simulink model "ds_modelica_weather"  (R2020a)
settings: Solver=ode1  StartTime=0.0  StopTime=Inf  FixedStep=0.001  RelTol=1e-3
PostLoadFcn:
  | if any(exist('dsrtsu_mdlpostloadfcn', 'file') ~= 0), dsrtsu_mdlpostloadfcn('Execute', bdroot); end
InitFcn:
  | , if any(exist('rtifpga_mdlclblib', 'file') ~= 0), rtifpga_mdlclblib('Init', bdroot); end,
  | , if any(exist('dsmpb_private', 'file') ~= 0), dsmpb_private('dsmpb_mdlclblib', 'Init', bdroot); end,
libraries: dsmpblib x1
PreSaveFcn:
  | , if any(exist('dsmpb_private', 'file') ~= 0), dsmpb_private('dsmpb_mdlclblib', 'PreSave', bdroot); end,
CloseFcn:
  | , if any(exist('dsmpb_private', 'file') ~= 0), dsmpb_private('dsmpb_mdlclblib', 'Close', bdroot); end,
settings Model: RTICANMMDATA=struct('GeneralSetupData',struct('modelroot','D:\github\dspace-modelica-example\dSpaceExample','generalsettings',struct('filesettings',struct('destfolder',struct('Name','RTICANMM_FILES','Check',1),'buildfolder',struct('Name','.','Check',1),'AbsDestfolder',struct('Name','D:\github\dspace-modelica-example\dSpaceExample\RTICANMM_FILES'),'AbsBuildfolder',struct('Name','D:\github\dspace-modelica-example\dSpaceExample'))),'options',struct('addpaths',1,'rmpaths',1,'addtrcexclusion',true,'cannavigator',struct('checkmonitoring',0),'show_usrtrc',0,'use_usrtrc',0),'advanced',struct('options',ones(1,100)),'MPSetup',{{}},'RTI',struct('Type','DSRT','Ver','4.3','Date','02-May-2020'),'modelname','ds_modelica_weather','block','ds_modelica_weather'))  DSRTSU_INTERNAL_RTIFPGA=160  DSMPB_ID_DATA={'121',struct('BlockId','15cad6c1-5c06-4fa3-8d72-980126a11d0f','SignalIds',{{'1464f171-9d95-458e-bcaf-80b82fdb8b87'}}),'122',struct('BlockId','3f54ef79-c7ab-4360-bc2a-717f94988ba9','SignalIds',{{'4ded6036-5f3c-446a-9a50-a2f43caa1de9'}}),'123',struct('BlockId','5b0f3eb3-8eee-4187-a879-1e3532fb32ad','SignalIds',{{'cf7abe49-a5c7-4834-bdd1-b99bcd3cf414'}}),'124',struct('BlockId','811b07df-2fcb-4c14-ad4d-f777e9630052','SignalIds',{{'eb3c2c6c-56b8-4259-a6b1-e5e06496ac5b'}}),'13',struct('BlockId','15cad6c1-5c06-4fa3-8d72-980126a11d0f','SignalIds',{{'1464f171-9d95-458e-bcaf-80b82fdb8b87'}}),'153',struct('BlockId','811b07df-2fcb-4c14-ad4d-f777e9630052','SignalIds',{{'eb3c2c6c-56b8-4259-a6b1-e5e06496ac5b'}})}  Creator=yangyang.fu  LastModifiedBy=yangyang.fu
settings OptimizationCC: BlockReduction=off  ConditionallyExecuteInputs=off  OptimizeBlockIOStorage=off  BufferReuse=off
settings DebuggingCC: TasksWithSamePriorityMsg=none
settings HardwareCC: ProdBitPerPointer=32  ProdBitPerSizeT=32  ProdBitPerPtrDiffT=32  ProdLargestAtomicInteger=Integer  ProdWordSize=32  ProdLongLongMode=on  ProdHWDeviceType=Custom Processor->Custom
settings ModelReferenceCC: EnableParallelModelReferenceBuilds=on
settings SFSimCC: MATLABDynamicMemAlloc=off
settings RTWCC: Description=dSPACE Run-Time Target (for VEOS on Windows and ConfigurationDesk)  SystemTargetFile=dsrt.tlc  GenCodeOnly=on  MakeCommand=make_dsrt  TemplateMakefile=dsrt_default_tmf  RTWVerbose=off  CustomInclude="\"C:\\Program Files\\Dymola 2021\\Source\" \"D:\\github\\dspace-modelica-example\\Libraries\\Buildings 7.0.0\\Resources\\C-Sources\""
settings STFCustomTargetCC: TargetLangStandard=C99 (ISO)  ParMdlRefBuildCompliant=on  SystemTargetFile=dsrt.tlc
settings GRTTargetCC: CompOptLevelCompliant=off  ConcurrentExecutionCompliant=off  CombineOutputUpdateFcns=off  MatFileLogging=off  CPPClassGenCompliant=off  UseToolchainInfoCompliant=off

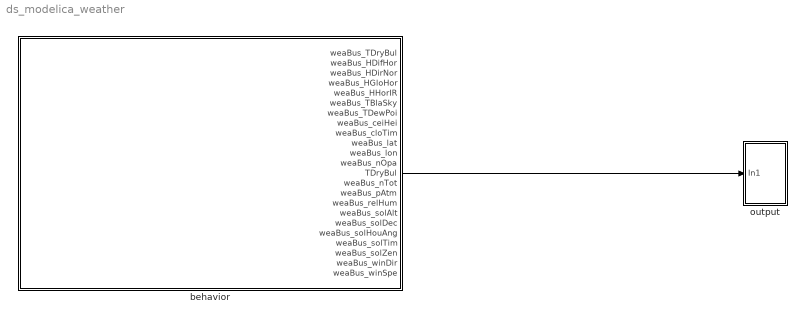
== system ds_modelica_weather ==
  behavior : Subsystem
  output : Subsystem
  wires:
  behavior/13(TDryBul) -> output/1(In1)

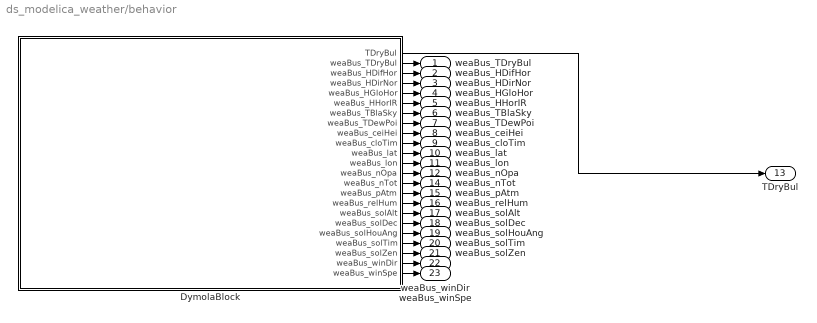
== system ds_modelica_weather/behavior ==
  DymolaBlock : Subsystem  Tag=19-Oct-2021 13:05:11#4854
      mask help:
      | Dymola block.
      | A dymola block allows acausal physical modeling.
      | See Dymola manual for usage.
      settings: CopyFcn=newDymolaGui('19-Oct-2021 13:05:11#4854','Copy');  DeleteFcn=if exist('newDymolaGui') newDymolaGui('ds_modelica_weather/behavior/DymolaBlock','Delete'); end;  NameChangeFcn=newDymolaGui('19-Oct-2021 13:05:11#4854','Copy');  OpenFcn=newDymolaGui('ds_modelica_weather/behavior/DymolaBlock','Init');
      mask Display: image(reshape([1;1;1;1;1;1;1;1;1;1;1;1;1;1;1;1;1;1;1;1;1;1;0;0;0;0;0;0;0;0;0;0;1;1;1;1;1;1;1;1;0;1;1;1;1;1;1;1;1;0;1;1;1;1;1;0;0;0;0;0;0;0;1;1;0;0;0;0;0;0;0;1;1;0;0;0;0;0;0;0;1;1;0;0;0;0;0;0;0;1;1;0;0;0;0;0;0;0;1;1;0;0;0;0;0;0;0;1;1;0;0;0;0;0;0;0;1;1;0;0;0;0;0;0;0;1;1;0;0;0;0;0;0;0;1;1;0;0;0;0;0;0;0;1;1;0;0;0;0;0;0;0;1;1;0;0;0;0;0;0;0;1;1;0;0;0;0;0;0;0;1;1;0;0;0;0;0;0;0;1;1;0;0;0;0;0;0;0;1;1;0;0;0;0;0;0;0;1;1;0;0;0;0;0;0;0;1;1;0;0;0;0;0;0;0;1;1;0;0;0;0;0;0;0;1;1;0;0;0;0;0;0;0;1;1;0;0;0;0;0;0;0;1;1;0;0;0;0;0;0;0;1;1;0;0;0;0;0;0;0;1;1;0;0;0;0;0;0;0;1;1;1;1;1;0;1;1;1;1;1;1;1;1;0;1;1;1;1;1;1;1;1;0;0;0;0;0;0;0;0;0;0;1;1;1;1;1;1;1;1;1;1;1;1;1;1;1;1;1;1;1;1;1;1;1;1;1;1;1;1;1;1;1;1;1;1;1;1;1;1;1;1;1;1;1;1;0;0;0;0;0;0;0;0;0;0;1;1;1;1;1;1;1;1;0;1;1;1;1;1;1;1;1;0;1;1;1;1;1;0;0;0;0;0;0;0;1;1;0;0;0;0;0;0;0;1;1;0;0;0;0;0;0;0;1;1;0;0;0;0;0;0;0;1;1;0;0;0;0;0;0;0;1;1;0;0;0;0;0;0;0;1;1;0;0;0;0;0;0;0;1;1;0;0;0;0;0;0;0;1;1;0;0;0;0;0;0;0;1;1;0;0;0;0;0;0;0;1;1;0;0;0;0;0;0;0;1;1;0;0;0;0;0;0;0;1;1;0;0;0;0;0;0;0;1;1;0;0;0;0;0;0;0;1;1;0;0;0;0;0;0;0;1;1;0;0;0;0;0;0;0;1;1;0;0;0;0;0;0;0;1;1;0;0;0;0;0;0;0;1;1;0;0;0;0;0;0;0;1;1;0;0;0;0;0;0;0;1;1;0;0;0;0;0;0;0;1;1;0;0;0;0;0;0;0;1;1;0;0;0;0;0;0;0;1;1;0;0;0;0;0;0;0;1;1;1;1;1;0;1;1;1;1;1;1;1;1;0;1;1;1;1;1;1;1;1;0;0;0;0;0;0;0;0;0;0;1;1;1;1;1;1;1;1;1;1;1;1;1;1;1;1;1;1;1;1;1;1;1;1;1;1;1;1;1;1;1;1;1;1;1;1;1;1;1;1;1;1;1;1;0;0;0;0;0;0;0;0;0;0;1;1;1;1;1;1;1;1;0;1;1;1;1;1;1;1;1;0;1;1;1;1;1;0;0;0;0;0;0;0;1;1;0;0;0;0;0;0;0;1;1;0;1;1;1;1;1;0;1;1;0;1;1;1;1;1;0;1;1;0;1;1;1;1;1;0;1;1;0;1;1;1;1;1;0;1;1;0;1;1;1;1;1;0;1;1;0;1;1;1;1;1;0;1;1;0;1;1;1;1;1;0;1;1;0;1;1;1;1;1;0;1;1;0;1;1;1;1;1;0;1;1;0;1;1;1;1;1;0;1;1;0;1;1;1;1;1;0;1;1;0;1;1;1;1;1;0;1;1;0;1;1;1;1;1;0;1;1;0;1;1;1;1;1;0;1;1;0;1;1;1;1;1;0;1;1;0;1;1;1;1;1;0;1;1;0;1;1;1;1;1;0;1;1;0;1;1;1;1;1;0;1;1;0;1;1;1;1;1;0;1;1;0;1;1;1;1;1;0;1;1;0;0;0;0;0;0;0;1;1;0;0;0;0;0;0;0;1;1;1;1;1;0;1;1;1;1;1;1;1;1;0;1;1;1;1;1;1;1;1;0;0;0;0;0;0;0;0;0;0;1;1;1;1;1;1;1;1;1;1;1;1;1;1;1;1;1;1;1;1;1;1],18,18,3),[.2,.2,.6,.6])
  weaBus_TDryBul : Outport
  weaBus_HDifHor : Outport  Port=2
  weaBus_HDirNor : Outport  Port=3
  weaBus_HGloHor : Outport  Port=4
  weaBus_HHorIR : Outport  Port=5
  weaBus_TBlaSky : Outport  Port=6
  weaBus_TDewPoi : Outport  Port=7
  weaBus_ceiHei : Outport  Port=8
  weaBus_cloTim : Outport  Port=9
  weaBus_lat : Outport  Port=10
  weaBus_lon : Outport  Port=11
  weaBus_nOpa : Outport  Port=12
  TDryBul : Outport  Port=13
  weaBus_nTot : Outport  Port=14
  weaBus_pAtm : Outport  Port=15
  weaBus_relHum : Outport  Port=16
  weaBus_solAlt : Outport  Port=17
  weaBus_solDec : Outport  Port=18
  weaBus_solHouAng : Outport  Port=19
  weaBus_solTim : Outport  Port=20
  weaBus_solZen : Outport  Port=21
  weaBus_winDir : Outport  Port=22
  weaBus_winSpe : Outport  Port=23
  wires:
  DymolaBlock/15(weaBus_pAtm) -> weaBus_pAtm/1
  DymolaBlock/14(weaBus_nTot) -> weaBus_nTot/1
  DymolaBlock/7(weaBus_TBlaSky) -> weaBus_TBlaSky/1
  DymolaBlock/21(weaBus_solZen) -> weaBus_solZen/1
  DymolaBlock/8(weaBus_TDewPoi) -> weaBus_TDewPoi/1
  DymolaBlock/11(weaBus_lat) -> weaBus_lat/1
  DymolaBlock/22(weaBus_winDir) -> weaBus_winDir/1
  DymolaBlock/5(weaBus_HGloHor) -> weaBus_HGloHor/1
  DymolaBlock/16(weaBus_relHum) -> weaBus_relHum/1
  DymolaBlock/10(weaBus_cloTim) -> weaBus_cloTim/1
  DymolaBlock/9(weaBus_ceiHei) -> weaBus_ceiHei/1
  DymolaBlock/13(weaBus_nOpa) -> weaBus_nOpa/1
  DymolaBlock/12(weaBus_lon) -> weaBus_lon/1
  DymolaBlock/1(TDryBul) -> TDryBul/1
  DymolaBlock/6(weaBus_HHorIR) -> weaBus_HHorIR/1
  DymolaBlock/17(weaBus_solAlt) -> weaBus_solAlt/1
  DymolaBlock/20(weaBus_solTim) -> weaBus_solTim/1
  DymolaBlock/18(weaBus_solDec) -> weaBus_solDec/1
  DymolaBlock/19(weaBus_solHouAng) -> weaBus_solHouAng/1
  DymolaBlock/23(weaBus_winSpe) -> weaBus_winSpe/1
  DymolaBlock/4(weaBus_HDirNor) -> weaBus_HDirNor/1
  DymolaBlock/2(weaBus_TDryBul) -> weaBus_TDryBul/1
  DymolaBlock/3(weaBus_HDifHor) -> weaBus_HDifHor/1

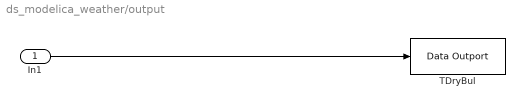
== system ds_modelica_weather/output ==
  In1 : Inport
  TDryBul : dsmpblib/Data Outport  Priority=-10000
      settings: SourceProductName=dSPACE Model Interface Blockset
  wires:
  In1/1 -> TDryBul/1

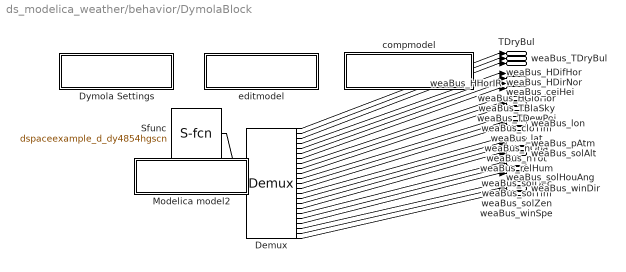
== system ds_modelica_weather/behavior/DymolaBlock ==
  Demux : Demux  Outputs=[1;1;1;1;1;1;1;1;1;1;1;1;1;1;1;1;1;1;1;1;1;1;1]
  Dymola Settings : Subsystem  mask{ModelName=dSpaceExample.Debug.WeatherReader, MoFileName=D:/github/dspace-modelica-example/dSpaceExample/Debug/WeatherReader.mo, dSpace=, BusConnector=[], ResultFile=[], ResultFileOnline=[], ResultDt=[], Libs=:, bigobj=[], ImportFolder=[], guimode=[], ModelName2=[], forRuntime=[], MEXLoad=[], omitDescription=[], ResultName=dspaceexample_d_dy4854hgscn}
      mask prompts: ModelName "Name of Dymola model"; MoFileName "File Name (including .mo)"; ResultFile "Create Result"; ResultFileOnline "Load result"; ResultDt "Result min dt"; Libs "Used Libraries"; bigobj "Compiler flag /bigobj"; ImportFolder "Import folder"; guimode "GUI mode flag"; ModelName2 "Model name for import mode"; forRuntime "Runtime export"; MEXLoad "Compiled S-function"; omitDescription "Omit description strings"; ResultName "Name of result file"
      mask Display: disp('Dymola Settings');
  Modelica model2 : Subsystem
      mask Display: disp('Change parameters');
  Sfunc : S-Function  Tag=4854hgscn  FunctionName=dspaceexample_d_dy4854hgscn  Parameters=[weaDat_pAtm;weaDat_TDryBul;weaDat_TDewPoi;weaDat_TBlaSky;weaDat_relHum;weaDat_winSpe;weaDat_winDir;weaDat_HInfHor;weaDat_ceiHei;weaDat_totSkyCov;weaDat_opaSkyCov;weaDat_datRea_verboseRead;weaDat_cheTemDryBul_TMin;weaDat_cheTemDryBul_TMax;weaDat_cheTemDewPoi_TMin;weaDat_cheTemDewPoi_TMax;weaDat_add30Min_k1;weaDat_add30Min_k2;weaDat_datRea30Min_verbos19;weaDat_cheTemBlaSky_TMin;weaDat_cheTemBlaSky_TMax],[]  PortCounts=[0;1]  SFunctionDeploymentMode=off  EnableBusSupport=off  mask{weaDat_pAtm=101325, weaDat_TDryBul=293.15, weaDat_TDewPoi=283.15, weaDat_TBlaSky=273.15, weaDat_relHum=0.5, weaDat_winSpe=1, weaDat_winDir=1, weaDat_HInfHor=0, weaDat_ceiHei=20000, weaDat_totSkyCov=0.5, weaDat_opaSkyCov=0.5, weaDat_datRea_verboseRead=0, weaDat_cheTemDryBul_TMin=203.15, weaDat_cheTemDryBul_TMax=343.15, weaDat_cheTemDewPoi_TMin=203.15, weaDat_cheTemDewPoi_TMax=343.15, weaDat_add30Min_k1=1, weaDat_add30Min_k2=1, weaDat_datRea30Min_verbos19=0, weaDat_cheTemBlaSky_TMin=0, weaDat_cheTemBlaSky_TMax=343.15}
      mask prompts: weaDat_pAtm "weaDat.pAtm"; weaDat_TDryBul "weaDat.TDryBul"; weaDat_TDewPoi "weaDat.TDewPoi"; weaDat_TBlaSky "weaDat.TBlaSky"; weaDat_relHum "weaDat.relHum"; weaDat_winSpe "weaDat.winSpe"; weaDat_winDir "weaDat.winDir"; weaDat_HInfHor "weaDat.HInfHor"; weaDat_ceiHei "weaDat.ceiHei"; weaDat_totSkyCov "weaDat.totSkyCov"; weaDat_opaSkyCov "weaDat.opaSkyCov"; weaDat_datRea_verboseRead "weaDat.datRea.verboseRead"; weaDat_cheTemDryBul_TMin "weaDat.cheTemDryBul.TMin"; weaDat_cheTemDryBul_TMax "weaDat.cheTemDryBul.TMax"; weaDat_cheTemDewPoi_TMin "weaDat.cheTemDewPoi.TMin"; weaDat_cheTemDewPoi_TMax "weaDat.cheTemDewPoi.TMax"; weaDat_add30Min_k1 "weaDat.add30Min.k1"; weaDat_add30Min_k2 "weaDat.add30Min.k2"; weaDat_datRea30Min_verbos19 "weaDat.datRea30Min.verboseRead"; weaDat_cheTemBlaSky_TMin "weaDat.cheTemBlaSky.TMin"; weaDat_cheTemBlaSky_TMax "weaDat.cheTemBlaSky.TMax"
      mask Display: image(imread('Dymola.bmp'))
  compmodel : Subsystem
      settings: OpenFcn=compileModelica('ds_modelica_weather/behavior/DymolaBlock');
      mask Display: disp('Compile Modelica model');
  editmodel : Subsystem
      settings: OpenFcn=editModelica('ds_modelica_weather/behavior/DymolaBlock');
      mask Display: disp('Edit Modelica model');
  TDryBul : Outport
  weaBus_TDryBul : Outport  Port=2
  weaBus_HDifHor : Outport  Port=3
  weaBus_HDirNor : Outport  Port=4
  weaBus_HGloHor : Outport  Port=5
  weaBus_HHorIR : Outport  Port=6
  weaBus_TBlaSky : Outport  Port=7
  weaBus_TDewPoi : Outport  Port=8
  weaBus_ceiHei : Outport  Port=9
  weaBus_cloTim : Outport  Port=10
  weaBus_lat : Outport  Port=11
  weaBus_lon : Outport  Port=12
  weaBus_nOpa : Outport  Port=13
  weaBus_nTot : Outport  Port=14
  weaBus_pAtm : Outport  Port=15
  weaBus_relHum : Outport  Port=16
  weaBus_solAlt : Outport  Port=17
  weaBus_solDec : Outport  Port=18
  weaBus_solHouAng : Outport  Port=19
  weaBus_solTim : Outport  Port=20
  weaBus_solZen : Outport  Port=21
  weaBus_winDir : Outport  Port=22
  weaBus_winSpe : Outport  Port=23
  wires:
  Sfunc/1 -> Demux/1
  Demux/1 -> TDryBul/1
  Demux/2 -> weaBus_TDryBul/1
  Demux/3 -> weaBus_HDifHor/1
  Demux/4 -> weaBus_HDirNor/1
  Demux/5 -> weaBus_HGloHor/1
  Demux/6 -> weaBus_HHorIR/1
  Demux/7 -> weaBus_TBlaSky/1
  Demux/8 -> weaBus_TDewPoi/1
  Demux/9 -> weaBus_ceiHei/1
  Demux/10 -> weaBus_cloTim/1
  Demux/11 -> weaBus_lat/1
  Demux/12 -> weaBus_lon/1
  Demux/13 -> weaBus_nOpa/1
  Demux/14 -> weaBus_nTot/1
  Demux/15 -> weaBus_pAtm/1
  Demux/16 -> weaBus_relHum/1
  Demux/17 -> weaBus_solAlt/1
  Demux/18 -> weaBus_solDec/1
  Demux/19 -> weaBus_solHouAng/1
  Demux/20 -> weaBus_solTim/1
  Demux/21 -> weaBus_solZen/1
  Demux/22 -> weaBus_winDir/1
  Demux/23 -> weaBus_winSpe/1

== system ds_modelica_weather/behavior/DymolaBlock/Dymola Settings ==

== system ds_modelica_weather/behavior/DymolaBlock/Modelica model2 ==

== system ds_modelica_weather/behavior/DymolaBlock/compmodel ==

== system ds_modelica_weather/behavior/DymolaBlock/editmodel ==
